simulink model "Grav_comp"  (R2015a)
settings: Solver=ode3  StartTime=0.0  StopTime=inf  FixedStep=1e-3  RelTol=1e-3
values from neighbouring files (symbols this model uses):
  conversion_V2mm = 17.8/(3540-260)    (= 0.00542682926829)    [Datasheet.m]    (also in setup.m)
libraries: PoliArd x6, simulink x2
settings Model: ExtModeTrigDuration=2  Creator=User  LastModifiedBy=User
settings OptimizationCC: OptimizeModelRefInitCode=on  LifeSpan=1
settings DebuggingCC: UnderspecifiedInitializationDetection=Classic  MergeDetectMultiDrivingBlocksExec=none
settings HardwareCC: ProdLargestAtomicInteger=Long  ProdLargestAtomicFloat=Double  ProdEndianess=LittleEndian  ProdHWDeviceType=ARM Compatible->ARM Cortex
settings RTWCC: SystemTargetFile=realtime.tlc  GenerateMakefile=off  TemplateMakefile=realtime.tmf  Description=Run on Target Hardware  RTWVerbose=off
settings ERTTargetCC: CombineOutputUpdateFcns=off  ExtModeTransport=3  ExtModeMexFile=ext_serial_win32_comm_rtt  ExtModeMexArgs=0 1 9600  ERTSrcFileBannerTemplate=realtime_code_template.cgt  ERTHdrFileBannerTemplate=realtime_code_template.cgt  ERTDataSrcFileTemplate=realtime_code_template.cgt  ERTDataHdrFileTemplate=realtime_code_template.cgt  ERTCustomFileTemplate=realtime_file_process.tlc

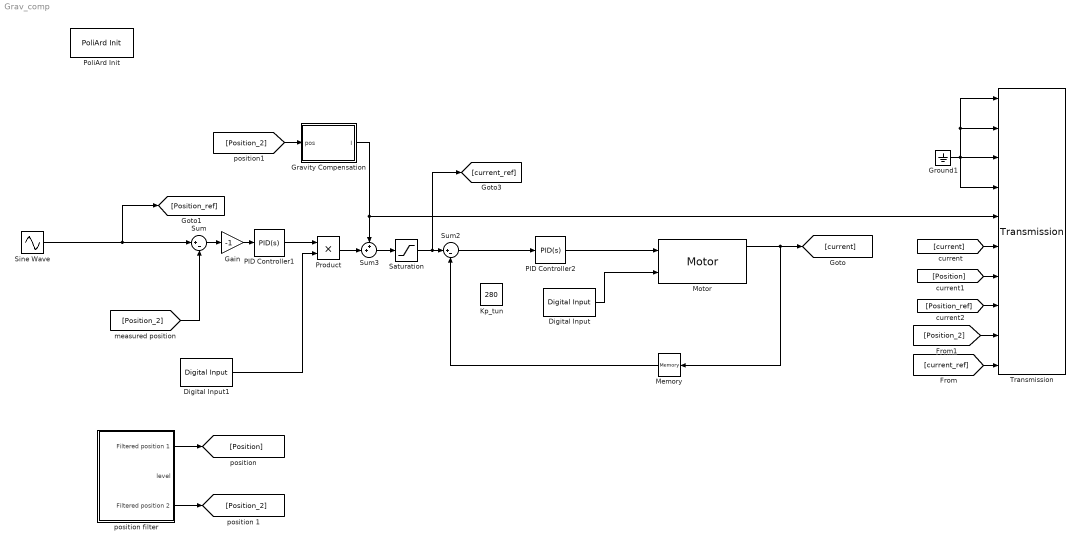
== system Grav_comp ==
  Digital Input : PoliArd/Digital Input  DI_pin=3  DIsample=-1
  Digital Input1 : PoliArd/Digital Input  DI_pin=2  DIsample=-1
  Gain : Gain  Gain=-1
  Gravity Compensation : MATLAB Function  TreatAsAtomicUnit=on
  Ground1 : Ground
  "Kp_tun " : Constant  Value=280
  Memory : Memory
  Motor : PoliArd/Motor  MotorID=2  DC_bus_mask=24  dt_mot=-1
  PID Controller1 : simulink/Continuous/PID Controller  Controller=PID  TimeDomain=Continuous-time  SampleTime=-1  IntegratorMethod=Forward Euler  FilterMethod=Forward Euler  Form=Parallel  UseFilter=on  ControllerParametersSource=internal  P=0.07  I=0.3  D=0.01  N=100  InitialConditionSource=internal  InitialConditionForIntegrator=0  InitialConditionForFilter=0  ExternalReset=none  LimitOutput=on  UpperSaturationLimit=0.4  LowerSaturationLimit=-0.4  LinearizeAsGain=on  AntiWindupMode=back-calculation  Kb=1  TrackingMode=off  Kt=1  PParamMin=[]  PParamMax=[]  IParamMin=[]  IParamMax=[]  DParamMin=[]  DParamMax=[]  NParamMin=[]  NParamMax=[]  KbParamMin=[]  KbParamMax=[]  KtParamMin=[]  KtParamMax=[]  POutMin=[]  POutMax=[]  IOutMin=[]  IOutMax=[]  DOutMin=[]  DOutMax=[]  NOutMin=[]  NOutMax=[]  KbOutMin=[]  KbOutMax=[]  KtOutMin=[]  KtOutMax=[]  IntegratorOutMin=[]  IntegratorOutMax=[]  FilterOutMin=[]  FilterOutMax=[]  SumOutMin=[]  SumOutMax=[]  SumI1OutMin=[]  SumI1OutMax=[]  SumI2OutMin=[]  SumI2OutMax=[]  SumI3OutMin=[]  SumI3OutMax=[]  SumDOutMin=[]  SumDOutMax=[]  SaturationOutMin=[]  SaturationOutMax=[]  IntegratorContinuousStateAttributes=''  IntegratorStateMustResolveToSignalObject=off  IntegratorRTWStateStorageClass=Auto  FilterContinuousStateAttributes=''  FilterStateMustResolveToSignalObject=off  FilterRTWStateStorageClass=Auto  DifferentiatorICPrevScaledInput=0  DifferentiatorOutMin=[]  DifferentiatorOutMax=[]
  PID Controller2 : simulink/Continuous/PID Controller  Controller=PID  TimeDomain=Continuous-time  SampleTime=-1  IntegratorMethod=Forward Euler  FilterMethod=Forward Euler  Form=Parallel  UseFilter=on  ControllerParametersSource=internal  P=24.75  I=697  D=0  N=0  InitialConditionSource=internal  InitialConditionForIntegrator=0  InitialConditionForFilter=0  ExternalReset=none  LimitOutput=on  UpperSaturationLimit=24  LowerSaturationLimit=-24  LinearizeAsGain=on  AntiWindupMode=none  Kb=1  TrackingMode=off  Kt=1  PParamMin=[]  PParamMax=[]  IParamMin=[]  IParamMax=[]  DParamMin=[]  DParamMax=[]  NParamMin=[]  NParamMax=[]  KbParamMin=[]  KbParamMax=[]  KtParamMin=[]  KtParamMax=[]  POutMin=[]  POutMax=[]  IOutMin=[]  IOutMax=[]  DOutMin=[]  DOutMax=[]  NOutMin=[]  NOutMax=[]  KbOutMin=[]  KbOutMax=[]  KtOutMin=[]  KtOutMax=[]  IntegratorOutMin=[]  IntegratorOutMax=[]  FilterOutMin=[]  FilterOutMax=[]  SumOutMin=[]  SumOutMax=[]  SumI1OutMin=[]  SumI1OutMax=[]  SumI2OutMin=[]  SumI2OutMax=[]  SumI3OutMin=[]  SumI3OutMax=[]  SumDOutMin=[]  SumDOutMax=[]  SaturationOutMin=[]  SaturationOutMax=[]  IntegratorContinuousStateAttributes=''  IntegratorStateMustResolveToSignalObject=off  IntegratorRTWStateStorageClass=Auto  FilterContinuousStateAttributes=''  FilterStateMustResolveToSignalObject=off  FilterRTWStateStorageClass=Auto  DifferentiatorICPrevScaledInput=0  DifferentiatorOutMin=[]  DifferentiatorOutMax=[]
  PoliArd Init : PoliArd/PoliArd Init
  Product : Product
  Saturation : Saturate  UpperLimit=10  LowerLimit=0
  Sine Wave : Sin  Amplitude=3.5  Bias=7.5  Frequency=6*pi  SampleTime=0
  Sum : Sum  Inputs=|+-
  Sum2 : Sum  Inputs=|+-
  Sum3 : Sum  Inputs=++|
  Transmission : PoliArd/Transmission  sample_freq=100  sig_to_send=6
  position filter : Subsystem
  wires:
  Motor/1 -> Memory/1, [current]
  position filter/1(Filtered position 1) -> [Position]
  [Position_2] -> Sum/2
  Sum2/1 -> PID Controller2/1
  Ground1/1 -> Transmission/4, Transmission/2, Transmission/1, Transmission/3
  Digital Input/1 -> Motor/2
  Memory/1 -> Sum2/2
  PID Controller2/1 -> Motor/1
  Sum3/1 -> Saturation/1
  [current] -> Transmission/6
  [Position] -> Transmission/7
  [Position_ref] -> Transmission/8
  [current_ref] -> Transmission/10
  Gravity Compensation/1(I) -> Transmission/5, Sum3/1
  Saturation/1 -> Sum2/1, [current_ref]
  Product/1 -> Sum3/2
  PID Controller1/1 -> Product/1
  Digital Input1/1 -> Product/2
  Sum/1 -> Gain/1
  Gain/1 -> PID Controller1/1
  Sine Wave/1 -> [Position_ref], Sum/1
  [Position_2] -> Gravity Compensation/1(pos)
  [Position_2] -> Transmission/9
  position filter/3(Filtered position 2) -> [Position_2]

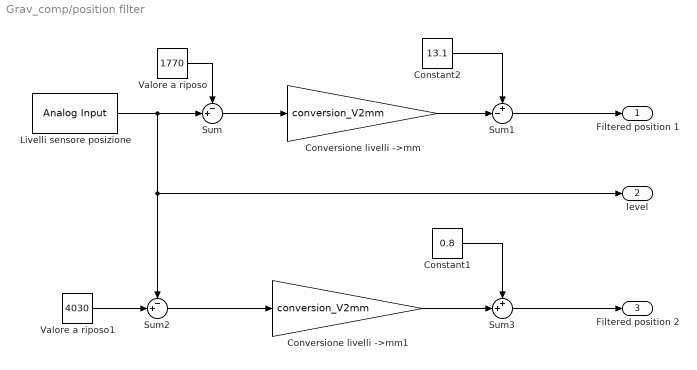
== system Grav_comp/position filter ==
  Constant1 : Constant  Value=0.8
  Constant2 : Constant  Value=13.1
  Conversione livelli ->mm : Gain  Gain=conversion_V2mm
  Conversione livelli ->mm1 : Gain  Gain=conversion_V2mm
  "Livelli sensore posizione " : PoliArd/Analog Input  AIpin_mask=2  AIsample=-1
  Sum : Sum  Inputs=-+|
  Sum1 : Sum  Inputs=+-|
  Sum2 : Sum  Inputs=-+|
  Sum3 : Sum  Inputs=++|
  Valore a riposo : Constant  Value=1770
  Valore a riposo1 : Constant  Value=4030
  Filtered position 1 : Outport
  "level " : Outport  Port=2
  Filtered position 2 : Outport  Port=3
  wires:
  "Livelli sensore posizione "/1 -> "level "/1, Sum2/1, Sum/2
  Sum/1 -> Conversione livelli ->mm/1
  Valore a riposo/1 -> Sum/1
  Conversione livelli ->mm/1 -> Sum1/2
  Constant2/1 -> Sum1/1
  Sum1/1 -> Filtered position 1/1
  Valore a riposo1/1 -> Sum2/2
  Sum2/1 -> Conversione livelli ->mm1/1
  Conversione livelli ->mm1/1 -> Sum3/2
  Sum3/1 -> Filtered position 2/1
  Constant1/1 -> Sum3/1

== matlab function Grav_comp/Gravity Compensation ==
  data: I output; pos input
function I = fcn(pos)
q=0.1115;
m = 0.1921;
I=pos*m+q;

end
